simulink model "SMC_POS_SMC_Att"  (R2024b)
settings: Solver=FixedStepDiscrete  StartTime=0.0  StopTime=45  FixedStep=1/250  RelTol=1e-3
values from neighbouring files (symbols this model uses):
  a1 = 3.5524    [Parameter_SMC.m]
  a2 = 10.000    (= 10)    [Parameter_SMC.m]
  a3 = 8.1910    (= 8.191)    [Parameter_SMC.m]
  a4 = 2.7640    (= 2.764)    [Parameter_SMC.m]
  b3 = 0.6373    [Parameter_SMC.m]
  b4 = 0.0223    [Parameter_SMC.m]
  b_1x = 0.7426    [Parameter_SMC.m]
  b_1y = 0.5930    (= 0.593)    [Parameter_SMC.m]
  b_2x = 1.4305    [Parameter_SMC.m]
  b_2y = 1.0895    [Parameter_SMC.m]
  c_x = 0.2871    [Parameter_SMC.m]
  c_y = 0.3867    [Parameter_SMC.m]
  epsilon_1_a = 0.5    [Parameter_SMC.m]
  epsilon_1_b = 0.5    [Parameter_SMC.m]
  epsilon_2 = 0.5    [Parameter_SMC.m]
  epsilon_2_b = 0.5    [Parameter_SMC.m]
  g = 9.81    [Parameter_SMC.m]
  Jx = 0.005    [Parameter_SMC.m]
  Jy = 0.005    [Parameter_SMC.m]
  Jz = 0.009    [Parameter_SMC.m]
  K1 = 0.01    [Parameter_SMC.m]
  k1 = 0.001    [Parameter_SMC.m]
  K2 = 0    [Parameter_SMC.m]
  k2 = a1    (= 3.5524)    [Parameter_SMC.m]
  k3 = 0.1    [Parameter_SMC.m]
  k4 = 0.5000    (= 0.5)    [Parameter_SMC.m]
  k5 = 0.0388    [Parameter_SMC.m]
  k6 = Jx * a3 / (l * sqrt(8) * Tmax)    [Parameter_SMC.m]
  k7 = 0.3147    [Parameter_SMC.m]
  k8 = a4 * Jz / (4 * Qmax)    (= 0.12438)    [Parameter_SMC.m]
  k_ob = 1    [Parameter_SMC.m]
  l = 0.33/2    (= 0.165)    [Parameter_SMC.m]
  m = 0.8    [Parameter_SMC.m]
  PWM_max = 2000    [Parameter_SMC.m]
  PWM_min = 1000    [Parameter_SMC.m]
  Qmax = 0.05    [Parameter_SMC.m]
  Tmax = 4    [Parameter_SMC.m]
undefined symbols (not defined in the file or in its folder): d_1_x, DiscIntNeverNeededParam, k_1_a, k_1_b, k_2_a, k_2_b, K_4, Q_max, T_max
libraries: simulink x13, slpidlib x3
(part 1 of 2)
settings Model: Creator=user  LastModifiedBy=user

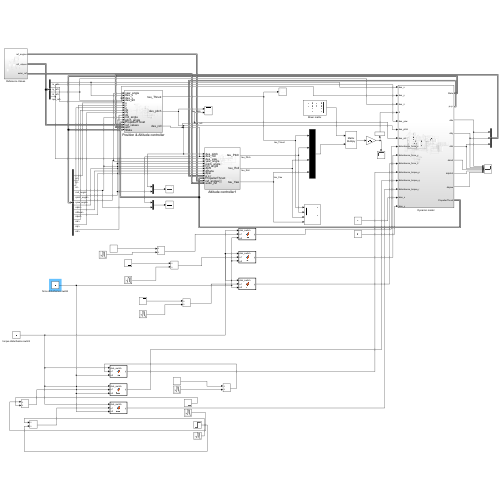
[thumbnail: Simulink's stored preview of the top-level diagram]
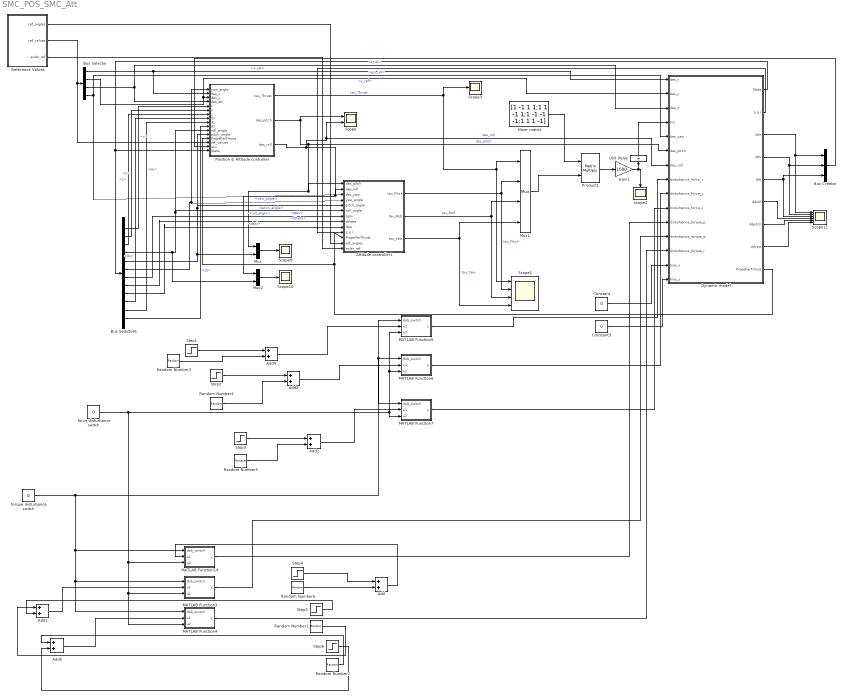
== system SMC_POS_SMC_Att ==
  Add{,1..5} (6 alike) : Sum
  Attitude controller1 : Subsystem
  Bus Creator : BusCreator  Inputs=3
  Bus Selector : BusSelector  OutputSignals=x_ref,y_ref,z_ref,psi_ref
  Bus Selector6 : BusSelector  OutputSignals=x,y,z,roll_angle,pitch_angle,yaw_angle,dphi,dtheta,dpsi,dx,dy,dz
  Constant : Constant  Value=0  SampleTime=-1
  Constant3 : Constant  Value=0  SampleTime=-1
  "Dynamic model " : Subsystem
  Gain1 : Gain  Gain=1000  OutDataTypeStr=double
  MATLAB Function14 : MATLAB Function  TreatAsAtomicUnit=on
  MATLAB Function3 : MATLAB Function  TreatAsAtomicUnit=on
  MATLAB Function4 : MATLAB Function  TreatAsAtomicUnit=on
  MATLAB Function5 : MATLAB Function  TreatAsAtomicUnit=on
  MATLAB Function6 : MATLAB Function  TreatAsAtomicUnit=on
  MATLAB Function7 : MATLAB Function  TreatAsAtomicUnit=on
  Mixer matrix : Constant  Value=[1 -1 1 1;1 1 -1 1;1 -1 -1 -1;1 1 1 -1]  OutDataTypeStr=Inherit: Inherit via back propagation
  Mux : Mux  Inputs=2
  Mux1 : Mux
  Mux2 : Mux  Inputs=2
  Position & Altitude controller : Subsystem
  Product1 : Product  Multiplication=Matrix(*)  RndMeth=Zero
  Random Number{1..6} (6 alike) : RandomNumber  Variance=0.1
  Reference Values : Subsystem
  Scope : Scope  NumInputPorts=2
  Scope1 : Scope  NumInputPorts=4
  Scope{2..3,9..10} (4 alike) : Scope
  Scope11 : Scope  NumInputPorts=6
  Step1 : Step  Time=0  After=15
  Step2 : Step  Time=0  After=-15
  Step3 : Step  Time=0  After=2
  Step4 : Step  Time=0
  Step5 : Step  Time=0  After=-0.5
  Step6 : Step  Time=0  After=5
  Unit Delay : UnitDelay  SampleTime=-1  HasFrameUpgradeWarning=on
  force disturbance switch : Constant  Value=0  SampleTime=-1
  torque disturbance switch : Constant  Value=0  SampleTime=-1
  wires:
  "Dynamic model "/5(ddz) -> Bus Creator/3, Scope11/3
  Constant3/1 -> "Dynamic model "/15(bias_y)
  Bus Selector6/12 -> Position & Altitude controller/10(dz)  "<dz>"
  "Dynamic model "/8(ddyaw) -> Scope11/6
  Product1/1 -> Gain1/1
  Mux/1 -> Scope9/1
  Mixer matrix/1 -> Product1/1
  Position & Altitude controller/2(des_pitch) -> Scope/1, Mux/1, Attitude controller1/1(des_pitch), "Dynamic model "/6(des_pitch)  "des_pitch"
  "Dynamic model "/2(p q r) -> Attitude controller1/10(p q r)
  "Dynamic model "/1(State) -> Bus Selector6/1, Position & Altitude controller/16(State)
  Bus Selector6/11 -> Position & Altitude controller/9(dy)  "<dy>"
  Attitude controller1/3(tau_Yaw) -> Mux1/4, Scope1/4  "tau_Yaw"
  Bus Selector6/2 -> Position & Altitude controller/6(y)  "<y>"
  "Dynamic model "/9(PropellerThrust) -> Position & Altitude controller/13(PropellerThrust), Attitude controller1/11(PropellerThrust)
  Attitude controller1/1(tau_Pitch) -> Mux1/2, Scope1/2  "tau_Pitch"
  Constant/1 -> "Dynamic model "/14(bias_x)
  "Dynamic model "/4(ddy) -> Bus Creator/2, Scope11/2
  Bus Selector6/1 -> Position & Altitude controller/5(x)  "<x>"
  Mux2/1 -> Scope10/1
  Bus Selector6/9 -> Attitude controller1/9(dpsi)  "<dpsi>"
  Bus Selector6/5 -> Position & Altitude controller/12(pitch_angle), Attitude controller1/5(pitch_angle), Mux/2  "<pitch_angle>"
  Gain1/1 -> Scope2/1, Unit Delay/1
  Bus Selector6/10 -> Position & Altitude controller/8(dx)  "<dx>"
  Bus Selector6/6 -> Position & Altitude controller/1(yaw_angle), Attitude controller1/4(yaw_angle)  "<yaw_angle>"
  Position & Altitude controller/1(tau_Thrust) -> Scope3/1, Mux1/1, Scope1/1  "tau_Thrust"
  Bus Selector6/4 -> Mux2/2, Position & Altitude controller/11(roll_angle), Attitude controller1/6(roll_angle)  "<roll_angle>"
  "Dynamic model "/6(ddroll) -> Scope11/4
  "Dynamic model "/7(ddpitch) -> Scope11/5
  Bus Selector6/8 -> Attitude controller1/8(dtheta)  "<dtheta>"
  Bus Selector6/7 -> Attitude controller1/7(dphi)  "<dphi>"
  Attitude controller1/2(tau_Roll) -> Mux1/3, Scope1/3  "tau_Roll"
  Position & Altitude controller/3(des_roll) -> Mux2/1, Attitude controller1/2(des_roll), "Dynamic model "/7(des_roll), Scope/2  "des_roll"
  "Dynamic model "/3(ddx) -> Bus Creator/1, Scope11/1
  Bus Selector6/3 -> Position & Altitude controller/7(z)  "<z>"
  Mux1/1 -> Product1/2
  Reference Values/2(ref_values) -> Position & Altitude controller/14(ref_values), Bus Selector/1
  Bus Selector/1 -> "Dynamic model "/1(des_x), Position & Altitude controller/2(des_x)  "<x_ref>"
  Bus Selector/2 -> "Dynamic model "/2(des_y), Position & Altitude controller/3(des_y)  "<y_ref>"
  Bus Selector/3 -> Position & Altitude controller/4(des_alt), "Dynamic model "/3(des_z)  "<z_ref>"
  Bus Selector/4 -> Attitude controller1/3(des_yaw), "Dynamic model "/5(des_yaw)  "<psi_ref>"
  Reference Values/1(ref_angles) -> Attitude controller1/12(ref_angles)
  Reference Values/3(euler_ref) -> Attitude controller1/13(euler_ref)
  Bus Creator/1 -> Position & Altitude controller/15(acc)
  Unit Delay/1 -> "Dynamic model "/4(In1)
  Random Number1/1 -> Add1/1
  Add4/1 -> MATLAB Function5/2(u1)
  torque disturbance switch/1 -> MATLAB Function5/1(dob_switch), MATLAB Function7/1(dob_switch), MATLAB Function6/1(dob_switch), MATLAB Function14/1(dob_switch), MATLAB Function4/1(dob_switch), MATLAB Function3/1(dob_switch)
  Step3/1 -> Add2/1
  Step6/1 -> Add5/2
  Step2/1 -> Add3/1
  Add2/1 -> MATLAB Function7/2(u1)
  Random Number2/1 -> Add5/1
  Step4/1 -> Add/1
  Random Number6/1 -> Add/2
  Add5/1 -> MATLAB Function4/2(u1)
  Random Number3/1 -> Add4/2
  Random Number4/1 -> Add3/2
  Add1/1 -> MATLAB Function3/2(u1)
  Random Number5/1 -> Add2/2
  force disturbance switch/1 -> MATLAB Function5/3(u2), MATLAB Function6/3(u2), MATLAB Function7/3(u2), MATLAB Function4/3(u2), MATLAB Function3/3(u2), MATLAB Function14/3(u2)
  Step5/1 -> Add1/2
  Add3/1 -> MATLAB Function6/2(u1)
  Step1/1 -> Add4/1
  Add/1 -> MATLAB Function14/2(u1)
  MATLAB Function5/1(y) -> "Dynamic model "/8(disturbance_force_x)
  MATLAB Function6/1(y) -> "Dynamic model "/9(disturbance_force_y)
  MATLAB Function7/1(y) -> "Dynamic model "/10(disturbance_force_z)
  MATLAB Function14/1(y) -> "Dynamic model "/11(disturbance_torque_p)
  MATLAB Function3/1(y) -> "Dynamic model "/12(disturbance_torque_q)
  MATLAB Function4/1(y) -> "Dynamic model "/13(disturbance_torque_r)

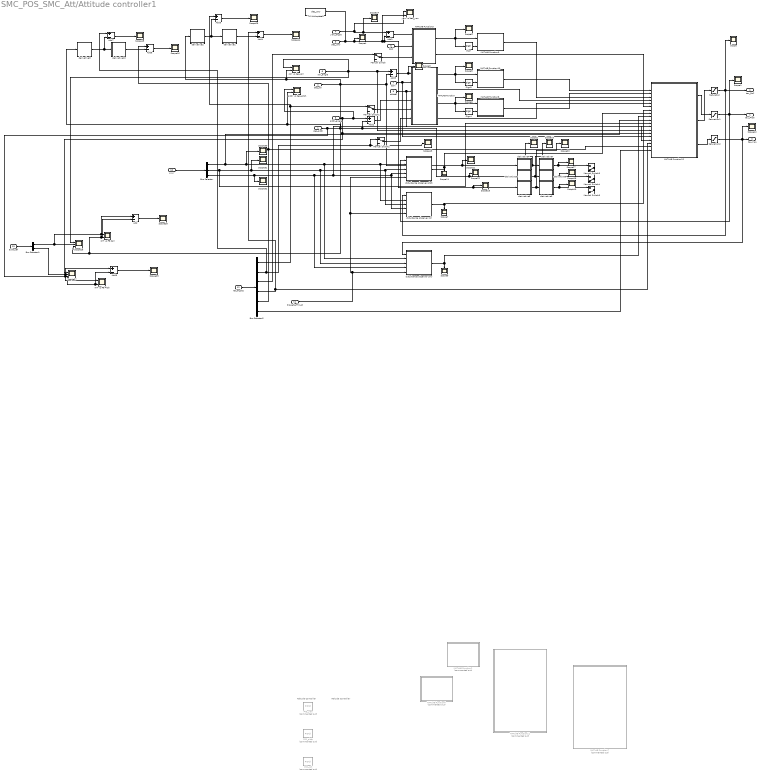
== system SMC_POS_SMC_Att/Attitude controller1 ==
  note: Attitude Controller
  note: Attitude Controller
  des_pitch : Inport
  des_roll : Inport  Port=2
  des_yaw : Inport  Port=3
  yaw_angle : Inport  Port=4
  pitch_angle : Inport  Port=5
  roll_angle : Inport  Port=6
  dphi : Inport  Port=7
  dtheta : Inport  Port=8
  dpsi : Inport  Port=9
  p q r : Inport  Port=10
  PropellerThrust : Inport  Port=11
  ref_angles : Inport  Port=12
  euler_ref : Inport  Port=13
  Add{,1..8} (9 alike) : Sum  Inputs=+-
  Bus Selector : BusSelector  OutputSignals=p,q,r
  Bus Selector1 : BusSelector  OutputSignals=phi_ref,theta_ref
  Bus Selector2 : BusSelector  OutputSignals=dphi_ref,dtheta_ref,dpsi_ref,ddphi_ref,ddtheta_ref,ddpsi_ref
  MATLAB Function : MATLAB Function  TreatAsAtomicUnit=on
  MATLAB Function10 : MATLAB Function  TreatAsAtomicUnit=on
  MATLAB Function11 : MATLAB Function  Commented=on  TreatAsAtomicUnit=on
  MATLAB Function12 : MATLAB Function  TreatAsAtomicUnit=on
  MATLAB Function3 : MATLAB Function  TreatAsAtomicUnit=on
  MATLAB Function5 : MATLAB Function  Commented=on  TreatAsAtomicUnit=on
  MATLAB Function6 : MATLAB Function  Commented=on  TreatAsAtomicUnit=on
  MATLAB Function7 : MATLAB Function  Commented=on  TreatAsAtomicUnit=on
  MATLAB Function8 : MATLAB Function  TreatAsAtomicUnit=on
  MATLAB Function9 : MATLAB Function  TreatAsAtomicUnit=on
  Manual Switch : ManualSwitch
  Manual Switch1 : ManualSwitch
  Manual Switch2 : ManualSwitch
  Manual Switch3 : ManualSwitch  CurrentSetting=0
  Manual Switch4 : ManualSwitch  CurrentSetting=0
  Manual Switch5 : ManualSwitch  CurrentSetting=0
  NIT vs FB Pitch : Scope  NumInputPorts=2
  NIT vs FB Roll : Scope  NumInputPorts=2
  PID_pitch : slpidlib/PID Controller  Commented=on  Controller=PID  Form=Parallel  TimeDomain=Continuous-time  UseExternalTs=off  SampleTime=-1  IntegratorMethod=Backward Euler  FilterMethod=Forward Euler  ControllerParametersSource=internal  P=0.027  I=0.005  UseKiTs=off  D=0.0145948093220339  UseExternalDerivativeSource=off  N=50  UseFilter=on  TunerSelectOption=Transfer Function Based (PID Tuner App)  InitialConditionSource=internal  InitialConditionForIntegrator=0  InitialConditionForFilter=0  DifferentiatorICPrevScaledInput=0  ExternalReset=level  TrackingMode=off  Kt=1  LimitOutput=on  SatLimitsSource=internal  UpperSaturationLimit=0.05  LowerSaturationLimit=-0.05  LinearizeAsGain=off  AntiWindupMode=none  Kb=1  LimitIntegrator=off  UpperIntegratorSaturationLimit=inf  LowerIntegratorSaturationLimit=-inf  POutMin=[]  POutMax=[]  IOutMin=[]  IOutMax=[]  DOutMin=[]  DOutMax=[]  NOutMin=[]  NOutMax=[]  SumOutMin=[]  SumOutMax=[]  SaturationOutMin=[]  SaturationOutMax=[]  PParamMin=[]  PParamMax=[]  IParamMin=[]  IParamMax=[]  DParamMin=[]  DParamMax=[]  NParamMin=[]  NParamMax=[]  KbParamMin=[]  KbParamMax=[]  KtParamMin=[]  KtParamMax=[]  KbOutMin=[]  KbOutMax=[]  KtOutMin=[]  KtOutMax=[]  IntegratorOutMin=[]  IntegratorOutMax=[]  FilterOutMin=[]  FilterOutMax=[]  SumI1OutMin=[]  SumI1OutMax=[]  SumI2OutMin=[]  SumI2OutMax=[]  SumI3OutMin=[]  SumI3OutMax=[]  SumI4OutMin=[]  SumI4OutMax=[]  SumDOutMin=[]  SumDOutMax=[]  DifferentiatorOutMin=[]  DifferentiatorOutMax=[]  FilterDiffOutCoefMin=[]  FilterDiffOutCoefMax=[]  ReciprocalOutMin=[]  ReciprocalOutMax=[]  SumDenOutMin=[]  SumDenOutMax=[]  SumNumOutMin=[]  SumNumOutMax=[]  DivideOutMin=[]  DivideOutMax=[]  UdiffTsProdOutMin=[]  UdiffTsProdOutMax=[]  NTsProdOutMin=[]  NTsProdOutMax=[]  UintegralTsProdOutMin=[]  UintegralTsProdOutMax=[]  UngainTsProdOutMin=[]  UngainTsProdOutMax=[]  ClampingZeroOutDataTypeStr=Inherit: Inherit via back propagation  ClampingZeroOutMin=[]  ClampingZeroOutMax=[]  FilterDenConstantOutDataTypeStr=Inherit: Inherit via back propagation  FilterDenConstantOutMin=[]  FilterDenConstantOutMax=[]  PCopyOutDataTypeStr=Inherit: Inherit via back propagation  PCopyOutMin=[]  PCopyOutMax=[]  NCopyOutDataTypeStr=Inherit: Inherit via back propagation  NCopyOutMin=[]  NCopyOutMax=[]  IntegratorContinuousStateAttributes=''  IntegratorStateMustResolveToSignalObject=off  IntegratorRTWStateStorageClass=Auto  FilterContinuousStateAttributes=''  FilterStateMustResolveToSignalObject=off  FilterRTWStateStorageClass=Auto  ParallelPVariant=InternalParameters  IdealPVariant=Disabled  IVariant=InternalParameters  DVariant=InternalParameters  IntegratorVariant=Continuous  SatVariant=Enabled  AWVariant=Passthrough  PCopyVariant=Disabled  TRVariant=Disabled  FdbkBlocksVariant=Forward  IdealPFdbkVariant=Disabled  SatFdbkVariant=Disabled  DerivativeFilterVariant=ContFilter  NVariant=InternalParameters  NCopyVariant=Disabled  FilterICVariant=InternalICsFilter  IntegratorICVariant=InternalICs  ExternalResetVariant=ExternalReset  TRSumVariant=Passthrough  SumFdbkVariant=Disabled  SumVariant=Sum_PID  TsampFilterVariant=InternalTs  TsampNgainVariant=Passthrough  TsampIntegralVariant=Disabled_SignalSpec  ExternalSaturationOutDataTypeStr=Inherit: Same as second input  DerivativeSourceVariant=ErrorSignal  PreIntVariant=InternalPreInt
  PID_roll : slpidlib/PID Controller  Commented=on  Controller=PID  Form=Parallel  TimeDomain=Continuous-time  UseExternalTs=off  SampleTime=-1  IntegratorMethod=Backward Euler  FilterMethod=Forward Euler  ControllerParametersSource=internal  P=0.03  I=0.005  UseKiTs=off  D=0.015  UseExternalDerivativeSource=off  N=100  UseFilter=on  TunerSelectOption=Transfer Function Based (PID Tuner App)  InitialConditionSource=internal  InitialConditionForIntegrator=0  InitialConditionForFilter=0  DifferentiatorICPrevScaledInput=0  ExternalReset=level  TrackingMode=off  Kt=1  LimitOutput=on  SatLimitsSource=internal  UpperSaturationLimit=0.05  LowerSaturationLimit=-0.05  LinearizeAsGain=off  AntiWindupMode=none  Kb=1  LimitIntegrator=off  UpperIntegratorSaturationLimit=inf  LowerIntegratorSaturationLimit=-inf  POutMin=[]  POutMax=[]  IOutMin=[]  IOutMax=[]  DOutMin=[]  DOutMax=[]  NOutMin=[]  NOutMax=[]  SumOutMin=[]  SumOutMax=[]  SaturationOutMin=[]  SaturationOutMax=[]  PParamMin=[]  PParamMax=[]  IParamMin=[]  IParamMax=[]  DParamMin=[]  DParamMax=[]  NParamMin=[]  NParamMax=[]  KbParamMin=[]  KbParamMax=[]  KtParamMin=[]  KtParamMax=[]  KbOutMin=[]  KbOutMax=[]  KtOutMin=[]  KtOutMax=[]  IntegratorOutMin=[]  IntegratorOutMax=[]  FilterOutMin=[]  FilterOutMax=[]  SumI1OutMin=[]  SumI1OutMax=[]  SumI2OutMin=[]  SumI2OutMax=[]  SumI3OutMin=[]  SumI3OutMax=[]  SumI4OutMin=[]  SumI4OutMax=[]  SumDOutMin=[]  SumDOutMax=[]  DifferentiatorOutMin=[]  DifferentiatorOutMax=[]  FilterDiffOutCoefMin=[]  FilterDiffOutCoefMax=[]  ReciprocalOutMin=[]  ReciprocalOutMax=[]  SumDenOutMin=[]  SumDenOutMax=[]  SumNumOutMin=[]  SumNumOutMax=[]  DivideOutMin=[]  DivideOutMax=[]  UdiffTsProdOutMin=[]  UdiffTsProdOutMax=[]  NTsProdOutMin=[]  NTsProdOutMax=[]  UintegralTsProdOutMin=[]  UintegralTsProdOutMax=[]  UngainTsProdOutMin=[]  UngainTsProdOutMax=[]  ClampingZeroOutDataTypeStr=Inherit: Inherit via back propagation  ClampingZeroOutMin=[]  ClampingZeroOutMax=[]  FilterDenConstantOutDataTypeStr=Inherit: Inherit via back propagation  FilterDenConstantOutMin=[]  FilterDenConstantOutMax=[]  PCopyOutDataTypeStr=Inherit: Inherit via back propagation  PCopyOutMin=[]  PCopyOutMax=[]  NCopyOutDataTypeStr=Inherit: Inherit via back propagation  NCopyOutMin=[]  NCopyOutMax=[]  IntegratorContinuousStateAttributes=''  IntegratorStateMustResolveToSignalObject=off  IntegratorRTWStateStorageClass=Auto  FilterContinuousStateAttributes=''  FilterStateMustResolveToSignalObject=off  FilterRTWStateStorageClass=Auto  ParallelPVariant=InternalParameters  IdealPVariant=Disabled  IVariant=InternalParameters  DVariant=InternalParameters  IntegratorVariant=Continuous  SatVariant=Enabled  AWVariant=Passthrough  PCopyVariant=Disabled  TRVariant=Disabled  FdbkBlocksVariant=Forward  IdealPFdbkVariant=Disabled  SatFdbkVariant=Disabled  DerivativeFilterVariant=ContFilter  NVariant=InternalParameters  NCopyVariant=Disabled  FilterICVariant=InternalICsFilter  IntegratorICVariant=InternalICs  ExternalResetVariant=ExternalReset  TRSumVariant=Passthrough  SumFdbkVariant=Disabled  SumVariant=Sum_PID  TsampFilterVariant=InternalTs  TsampNgainVariant=Passthrough  TsampIntegralVariant=Disabled_SignalSpec  ExternalSaturationOutDataTypeStr=Inherit: Same as second input  DerivativeSourceVariant=ErrorSignal  PreIntVariant=InternalPreInt
  PID_yaw : slpidlib/PID Controller  Commented=on  Controller=PID  Form=Parallel  TimeDomain=Continuous-time  UseExternalTs=off  SampleTime=-1  IntegratorMethod=Backward Euler  FilterMethod=Forward Euler  ControllerParametersSource=internal  P=0.08024000000000001  I=0.005  UseKiTs=off  D=0.075  UseExternalDerivativeSource=off  N=100  UseFilter=on  TunerSelectOption=Transfer Function Based (PID Tuner App)  InitialConditionSource=internal  InitialConditionForIntegrator=0  InitialConditionForFilter=0  DifferentiatorICPrevScaledInput=0  ExternalReset=level  TrackingMode=off  Kt=1  LimitOutput=on  SatLimitsSource=internal  UpperSaturationLimit=0.1  LowerSaturationLimit=-0.1  LinearizeAsGain=off  AntiWindupMode=none  Kb=1  LimitIntegrator=off  UpperIntegratorSaturationLimit=inf  LowerIntegratorSaturationLimit=-inf  POutMin=[]  POutMax=[]  IOutMin=[]  IOutMax=[]  DOutMin=[]  DOutMax=[]  NOutMin=[]  NOutMax=[]  SumOutMin=[]  SumOutMax=[]  SaturationOutMin=[]  SaturationOutMax=[]  PParamMin=[]  PParamMax=[]  IParamMin=[]  IParamMax=[]  DParamMin=[]  DParamMax=[]  NParamMin=[]  NParamMax=[]  KbParamMin=[]  KbParamMax=[]  KtParamMin=[]  KtParamMax=[]  KbOutMin=[]  KbOutMax=[]  KtOutMin=[]  KtOutMax=[]  IntegratorOutMin=[]  IntegratorOutMax=[]  FilterOutMin=[]  FilterOutMax=[]  SumI1OutMin=[]  SumI1OutMax=[]  SumI2OutMin=[]  SumI2OutMax=[]  SumI3OutMin=[]  SumI3OutMax=[]  SumI4OutMin=[]  SumI4OutMax=[]  SumDOutMin=[]  SumDOutMax=[]  DifferentiatorOutMin=[]  DifferentiatorOutMax=[]  FilterDiffOutCoefMin=[]  FilterDiffOutCoefMax=[]  ReciprocalOutMin=[]  ReciprocalOutMax=[]  SumDenOutMin=[]  SumDenOutMax=[]  SumNumOutMin=[]  SumNumOutMax=[]  DivideOutMin=[]  DivideOutMax=[]  UdiffTsProdOutMin=[]  UdiffTsProdOutMax=[]  NTsProdOutMin=[]  NTsProdOutMax=[]  UintegralTsProdOutMin=[]  UintegralTsProdOutMax=[]  UngainTsProdOutMin=[]  UngainTsProdOutMax=[]  ClampingZeroOutDataTypeStr=Inherit: Inherit via back propagation  ClampingZeroOutMin=[]  ClampingZeroOutMax=[]  FilterDenConstantOutDataTypeStr=Inherit: Inherit via back propagation  FilterDenConstantOutMin=[]  FilterDenConstantOutMax=[]  PCopyOutDataTypeStr=Inherit: Inherit via back propagation  PCopyOutMin=[]  PCopyOutMax=[]  NCopyOutDataTypeStr=Inherit: Inherit via back propagation  NCopyOutMin=[]  NCopyOutMax=[]  IntegratorContinuousStateAttributes=''  IntegratorStateMustResolveToSignalObject=off  IntegratorRTWStateStorageClass=Auto  FilterContinuousStateAttributes=''  FilterStateMustResolveToSignalObject=off  FilterRTWStateStorageClass=Auto  ParallelPVariant=InternalParameters  IdealPVariant=Disabled  IVariant=InternalParameters  DVariant=InternalParameters  IntegratorVariant=Continuous  SatVariant=Enabled  AWVariant=Passthrough  PCopyVariant=Disabled  TRVariant=Disabled  FdbkBlocksVariant=Forward  IdealPFdbkVariant=Disabled  SatFdbkVariant=Disabled  DerivativeFilterVariant=ContFilter  NVariant=InternalParameters  NCopyVariant=Disabled  FilterICVariant=InternalICsFilter  IntegratorICVariant=InternalICs  ExternalResetVariant=ExternalReset  TRSumVariant=Passthrough  SumFdbkVariant=Disabled  SumVariant=Sum_PID  TsampFilterVariant=InternalTs  TsampNgainVariant=Passthrough  TsampIntegralVariant=Disabled_SignalSpec  ExternalSaturationOutDataTypeStr=Inherit: Same as second input  DerivativeSourceVariant=ErrorSignal  PreIntVariant=InternalPreInt
  Saturation : Saturate  UpperLimit=0.05  LowerLimit=-0.05
  Saturation1 : Saturate  UpperLimit=0.05  LowerLimit=-0.05
  Saturation2 : Saturate  UpperLimit=0.1  LowerLimit=-0.1
  Scope{,1..25,28..32} (31 alike) : Scope
  Scope26 : Scope  NumInputPorts=3
  Scope27 : Scope  NumInputPorts=3
  Sign : Signum
  Sign4 : Signum
  Sign5 : Signum
  To Workspace3 : ToWorkspace  VariableName=des_yaw  SampleTime=-1
      settings: Save2DSignal=2-D array (concatenate along first dimension)
  derivative1 : Subsystem
  derivative10 : Subsystem
  derivative2 : Subsystem
  derivative3 : Subsystem
  derivative4 : Subsystem
  derivative5 : Subsystem
  derivative6 : Subsystem
  derivative7 : Subsystem
  derivative8 : Subsystem
  derivative9 : Subsystem
  disturbance observer pitch : Subsystem
  disturbance observer roll : Subsystem
  disturbance observer yaw : Subsystem
  pitch vs des_pitch : Scope  NumInputPorts=2
  roll vs des_roll : Scope  NumInputPorts=2
  yaw vs des_yaw : Scope  NumInputPorts=2
  tau_Pitch : Outport
  tau_Roll : Outport  Port=2
  tau_Yaw : Outport  Port=3
  wires:
  yaw_angle/1 -> Scope24/1, Add1/1, yaw vs des_yaw/1  "yaw_angle"
  des_yaw/1 -> To Workspace3/1, Scope4/1, yaw vs des_yaw/2, Scope23/1, derivative6/1(In1), Add1/2  "des_yaw"
  Saturation/1 -> Scope/1, tau_Roll/1, disturbance observer roll/1(tau_Roll)
  Saturation2/1 -> Scope12/1, disturbance observer yaw/1(tau_Yaw), tau_Yaw/1
  Add1/1 -> MATLAB Function3/1(error)  "yaw_error"
  MATLAB Function/2(error_dphi) -> MATLAB Function12/4(error_dphi)
  MATLAB Function/1(s_phi) -> Scope5/1, Sign5/1, MATLAB Function10/1(s)
  MATLAB Function/4(error_dtheta) -> MATLAB Function12/5(error_dtheta)
  MATLAB Function/3(s_theta) -> Scope6/1, Sign4/1, MATLAB Function8/1(s)
  dtheta/1 -> MATLAB Function12/16(dtheta), MATLAB Function/3(dtheta)
  dphi/1 -> MATLAB Function12/15(dphi), MATLAB Function/2(dphi)
  Add3/1 -> Scope8/1, MATLAB Function/1(error_phi)  "roll_error"
  Add2/1 -> MATLAB Function/4(error_theta)  "pitch_error"
  MATLAB Function3/2(error_dpsi) -> MATLAB Function12/6(error_dpsi)
  MATLAB Function3/1(s_psi) -> Scope3/1, Sign/1, MATLAB Function9/1(s)
  dpsi/1 -> MATLAB Function3/2(dpsi)
  p q r/1 -> Bus Selector/1
  Bus Selector/1 -> MATLAB Function12/10(p), Scope30/1, disturbance observer roll/2("p "), disturbance observer pitch/2("p "), disturbance observer yaw/2("p ")  "<p>"
  Bus Selector/2 -> disturbance observer pitch/3(q), disturbance observer roll/3(q), disturbance observer yaw/3(q), Scope31/1, MATLAB Function12/11(q)  "<q>"
  Bus Selector/3 -> MATLAB Function12/12(r), disturbance observer pitch/4(r), disturbance observer roll/4(r), disturbance observer yaw/4(r), Scope32/1  "<r>"
  disturbance observer pitch/1(d_ob) -> MATLAB Function12/8(d_ob_theta), Scope11/1
  disturbance observer roll/1(d_ob) -> MATLAB Function12/7(d_ob_phi), Scope7/1
  disturbance observer yaw/1(d_ob) -> Scope9/1, MATLAB Function12/9(d_ob_psi)
  Manual Switch/1 -> MATLAB Function3/3(des_dpsi)
  Manual Switch1/1 -> MATLAB Function/5(des_dphi)
  Manual Switch2/1 -> MATLAB Function/6(des_dtheta)
  Saturation1/1 -> disturbance observer pitch/1(tau_Pitch), tau_Pitch/1, Scope1/1
  Sign/1 -> MATLAB Function9/2(sgn)
  Sign4/1 -> MATLAB Function8/2(sgn)
  Sign5/1 -> MATLAB Function10/2(sgn)
  MATLAB Function10/1(sat_phi) -> MATLAB Function12/1(sat_phi)
  MATLAB Function8/1(sat_theta) -> MATLAB Function12/2(sat_theta)
  MATLAB Function9/1(sat_psi) -> MATLAB Function12/3(sat_psi)
  derivative4/1(Out1) -> Scope2/1, derivative7/1(In1)
  derivative5/1(Out1) -> Scope10/1, derivative8/1(In1)
  derivative6/1(Out1) -> Scope20/1, derivative9/1(In1)
  derivative7/1(Out1) -> Scope17/1, Manual Switch3/1
  derivative8/1(Out1) -> Scope18/1, Manual Switch4/1
  derivative9/1(Out1) -> Scope19/1, Manual Switch5/1
  MATLAB Function12/3(tau_yaw) -> Saturation2/1
  MATLAB Function12/1(tau_pitch) -> Saturation1/1
  MATLAB Function12/2(tau_roll) -> Saturation/1
  PropellerThrust/1 -> disturbance observer yaw/5(PropellerThrust), disturbance observer pitch/5(PropellerThrust), disturbance observer roll/5(PropellerThrust)
  ref_angles/1 -> Bus Selector2/1
  Bus Selector2/1 -> Add5/1, Manual Switch1/1  "<dphi_ref>"
  Bus Selector2/3 -> Manual Switch/1  "<dpsi_ref>"
  Bus Selector2/6 -> MATLAB Function12/19(des_ddpsi)  "<ddpsi_ref>"
  derivative3/1(Out1) -> Add7/2, derivative10/1(des_roll)  "d_theta_des"
  Add4/1 -> Scope14/1  "dd_phi ref-des"
  Add7/1 -> Scope15/1  "d_theta ref-des"
  derivative2/1(Out1) -> Add5/2, derivative1/1(des_roll)  "d_phi_des"
  derivative1/1(Out1) -> Add4/2  "dd_phi_des"
  Bus Selector2/2 -> Add7/1, Manual Switch2/1, Scope13/1  "<dtheta_ref>"
  Add5/1 -> Scope25/1  "d_phi ref-des"
  Bus Selector2/4 -> Add4/1, MATLAB Function12/17(des_ddphi)  "<ddphi_ref>"
  derivative10/1(Out1) -> Add6/2  "dd_theta_des"
  Add6/1 -> Scope16/1  "dd_theta ref-des"
  Bus Selector2/5 -> Add6/1, MATLAB Function12/18(des_ddtheta)  "<ddtheta_ref>"
  euler_ref/1 -> Bus Selector1/1
  pitch_angle/1 -> pitch vs des_pitch/1, Add2/1, Scope27/1, MATLAB Function12/14(theta)  "pitch_angle"
  Bus Selector1/1 -> Scope26/2, Add/1, NIT vs FB Roll/1  "<phi_ref>"
  Bus Selector1/2 -> NIT vs FB Pitch/1, Scope27/2, Add8/1  "<theta_ref>"
  roll_angle/1 -> roll vs des_roll/1, Scope26/1, MATLAB Function12/13(phi), Add3/1  "roll _angle"
  des_pitch/1 -> Add8/2, NIT vs FB Pitch/2, Scope27/3, derivative3/1(des_roll), pitch vs des_pitch/2, Scope22/1, derivative5/1(In1), Add2/2  "des_pitch"
  des_roll/1 -> Add/2, NIT vs FB Roll/2, Scope26/3, derivative2/1(des_roll), roll vs des_roll/2, Scope21/1, derivative4/1(In1), Add3/2  "des_roll"
  Add/1 -> Scope28/1  "NIT - FB Roll"
  Add8/1 -> Scope29/1  "NIT - FB Pitch"

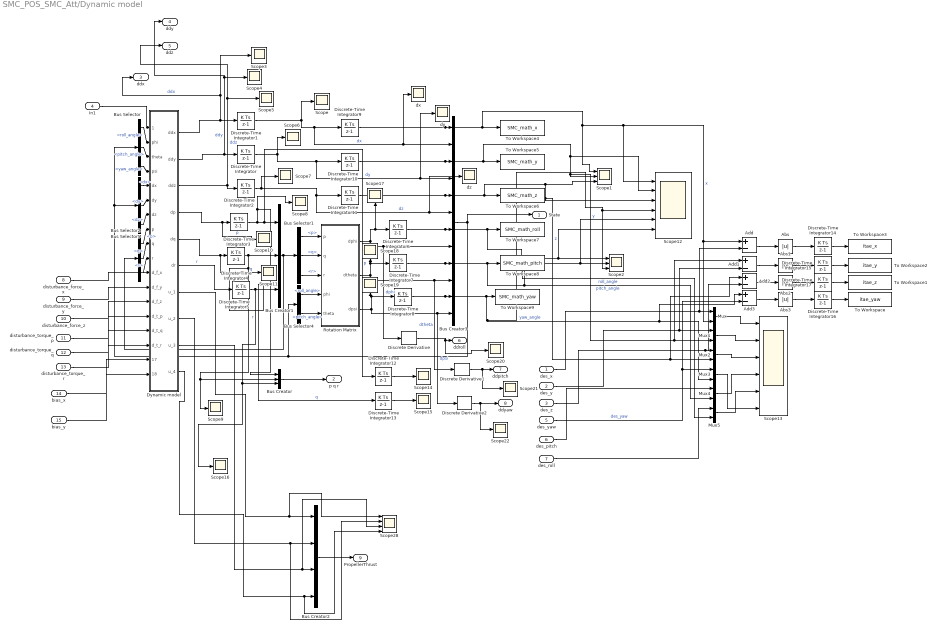
== system SMC_POS_SMC_Att/Dynamic model  ==
  des_x : Inport
  des_y : Inport  Port=2
  des_z : Inport  Port=3
  In1 : Inport  Port=4
  des_yaw : Inport  Port=5
  des_pitch : Inport  Port=6
  des_roll : Inport  Port=7
  disturbance_force_x : Inport  Port=8
  disturbance_force_y : Inport  Port=9
  disturbance_force_z : Inport  Port=10
  disturbance_torque_p : Inport  Port=11
  disturbance_torque_q : Inport  Port=12
  disturbance_torque_r : Inport  Port=13
  bias_x : Inport  Port=14
  bias_y : Inport  Port=15
  Abs{,1..3} (4 alike) : Abs  SaturateOnIntegerOverflow=off
  Add{,1..3} (4 alike) : Sum  Inputs=+-
  Bus Creator : BusCreator  Inputs=3
  Bus Creator1 : BusCreator  Inputs=3
  Bus Creator2 : BusCreator  Inputs=4
  Bus Creator3 : BusCreator  Inputs=12
  Bus Selector : BusSelector  OutputSignals=roll_angle,pitch_angle,yaw_angle
  Bus Selector1 : BusSelector  OutputSignals=p,q,r
  Bus Selector2 : BusSelector  OutputSignals=p,q,r
  Bus Selector4 : BusSelector  OutputSignals=roll_angle,pitch_angle
  Bus Selector5 : BusSelector  OutputSignals=dx,dy,dz
  Discrete Derivative : simulink/Discrete/Discrete Derivative  gainval=1.0  ICPrevScaledInput=0.0  OutMin=[]  OutMax=[]  OutDataType=fixdt(1, 16)  OutScaling=2^-10  DoSatur=off
  Discrete Derivative1 : simulink/Discrete/Discrete Derivative  gainval=1.0  ICPrevScaledInput=0.0  OutMin=[]  OutMax=[]  OutDataType=fixdt(1, 16)  OutScaling=2^-10  DoSatur=off
  Discrete Derivative2 : simulink/Discrete/Discrete Derivative  gainval=1.0  ICPrevScaledInput=0.0  OutMin=[]  OutMax=[]  OutDataType=fixdt(1, 16)  OutScaling=2^-10  DoSatur=off
  Discrete-Time Integrator{,1..17} (18 alike) : DiscreteIntegrator  SampleTime=-1  ICPrevOutput=DiscIntNeverNeededParam  ICPrevScaledInput=DiscIntNeverNeededParam
  Dynamic model : MATLAB Function  TreatAsAtomicUnit=on
  Mux{,1..5} (6 alike) : Mux  Inputs=2
  Rotation Matrix : MATLAB Function  TreatAsAtomicUnit=on
  Scope{,3..11,14..22} (19 alike) : Scope
  Scope1 : Scope  NumInputPorts=3
  Scope12 : Scope  NumInputPorts=6
  Scope13 : Scope  NumInputPorts=6
  Scope2 : Scope  NumInputPorts=3
  Scope28 : Scope  NumInputPorts=4
  To Workspace : ToWorkspace  VariableName=itae_yaw  SampleTime=-1
      settings: Save2DSignal=2-D array (concatenate along first dimension)
  To Workspace1 : ToWorkspace  VariableName=itae_z  SampleTime=-1
      settings: Save2DSignal=2-D array (concatenate along first dimension)
  To Workspace2 : ToWorkspace  VariableName=itae_y  SampleTime=-1
      settings: Save2DSignal=2-D array (concatenate along first dimension)
  To Workspace3 : ToWorkspace  VariableName=itae_x  SampleTime=-1
      settings: Save2DSignal=2-D array (concatenate along first dimension)
  To Workspace4 : ToWorkspace  VariableName=SMC_math_x  SampleTime=-1
      settings: Save2DSignal=2-D array (concatenate along first dimension)
  To Workspace5 : ToWorkspace  VariableName=SMC_math_y  SampleTime=-1
      settings: Save2DSignal=2-D array (concatenate along first dimension)
  To Workspace6 : ToWorkspace  VariableName=SMC_math_z  SampleTime=-1
      settings: Save2DSignal=2-D array (concatenate along first dimension)
  To Workspace7 : ToWorkspace  VariableName=SMC_math_roll  SampleTime=-1
      settings: Save2DSignal=2-D array (concatenate along first dimension)
  To Workspace8 : ToWorkspace  VariableName=SMC_math_pitch  SampleTime=-1
      settings: Save2DSignal=2-D array (concatenate along first dimension)
  To Workspace9 : ToWorkspace  VariableName=SMC_math_yaw  SampleTime=-1
      settings: Save2DSignal=2-D array (concatenate along first dimension)
  dx : Scope
  dy : Scope
  dz : Scope
  State : Outport
  p q r : Outport  Port=2
  ddx : Outport  Port=3
  ddy : Outport  Port=4
  ddz : Outport  Port=5
  ddroll : Outport  Port=6
  ddpitch : Outport  Port=7
  ddyaw : Outport  Port=8
  PropellerThrust : Outport  Port=9
  wires:
  Discrete-Time Integrator2/1 -> Scope7/1, Discrete-Time Integrator11/1, dz/1, Bus Creator3/6  "dz"
  Bus Selector4/1 -> Rotation Matrix/4(phi)  "<roll_angle>"
  Bus Selector5/1 -> Dynamic model/5(dx)  "<dx>"
  Dynamic model/3(ddz) -> Discrete-Time Integrator2/1, Scope5/1, ddz/1  "ddz"
  Bus Selector5/2 -> Dynamic model/6(dy)  "<dy>"
  Bus Selector1/2 -> Rotation Matrix/2(q)  "<q>"
  Bus Selector1/3 -> Rotation Matrix/3(r)  "<r>"
  Discrete-Time Integrator/1 -> Scope6/1, Discrete-Time Integrator10/1, dy/1, Bus Creator3/4  "dy"
  Dynamic model/5(dq) -> Scope11/1, Discrete-Time Integrator4/1  "q"
  Dynamic model/4(dp) -> Scope10/1, Discrete-Time Integrator3/1  "p"
  Rotation Matrix/3(dpsi) -> Scope19/1, Discrete-Time Integrator8/1, Discrete Derivative2/1, Bus Creator3/12  "dpsi"
  Dynamic model/1(ddx) -> Discrete-Time Integrator1/1, Scope3/1, ddx/1  "ddx"
  Bus Selector/1 -> Dynamic model/2(phi)  "<roll_angle>"
  Bus Selector2/1 -> Dynamic model/8(p)  "<p>"
  Dynamic model/6(dr) -> Discrete-Time Integrator5/1  "r"
  Dynamic model/2(ddy) -> Discrete-Time Integrator/1, Scope4/1, ddy/1  "ddy"
  Bus Selector2/3 -> Dynamic model/10(r)  "<r>"
  In1/1 -> Dynamic model/1(channel)
  Bus Selector4/2 -> Rotation Matrix/5(theta)  "<pitch_angle>"
  Bus Selector5/3 -> Dynamic model/7(dz)  "<dz>"
  Bus Creator1/1 -> Bus Selector1/1, Bus Selector2/1
  Bus Selector/2 -> Dynamic model/3(theta)  "<pitch_angle>"
  Bus Selector/3 -> Dynamic model/4(psi)  "<yaw_angle>"
  Bus Selector1/1 -> Rotation Matrix/1(p)  "<p>"
  Bus Selector2/2 -> Dynamic model/9(q)  "<q>"
  Rotation Matrix/1(dphi) -> Scope17/1, Discrete-Time Integrator6/1, Bus Creator3/8, Discrete Derivative/1  "dphi"
  Discrete-Time Integrator1/1 -> Scope/1, Discrete-Time Integrator9/1, dx/1, Bus Creator3/2  "dx"
  Bus Creator3/1 -> State/1, Bus Selector4/1, Bus Selector5/1, Bus Selector/1
  Rotation Matrix/2(dtheta) -> Scope18/1, Discrete-Time Integrator7/1, Discrete Derivative1/1, Bus Creator3/10  "dtheta"
  Mux/1 -> Scope13/1
  des_x/1 -> Add/2, Mux/1
  Mux1/1 -> Scope13/2
  des_y/1 -> Add1/2, Mux1/1
  des_z/1 -> Add2/2, Mux2/1
  des_yaw/1 -> Add3/2, Mux3/1  "des_yaw"
  des_pitch/1 -> Mux4/1
  des_roll/1 -> Mux5/1
  Mux2/1 -> Scope13/3
  Mux3/1 -> Scope13/6
  Mux4/1 -> Scope13/4
  Mux5/1 -> Scope13/5
  Bus Creator/1 -> p q r/1
  Discrete-Time Integrator3/1 -> Scope8/1, Bus Creator/1, Discrete-Time Integrator12/1, Bus Creator1/1  "p"
  Discrete-Time Integrator4/1 -> Discrete-Time Integrator13/1, Scope9/1, Bus Creator/2, Bus Creator1/2  "q"
  Add/1 -> Abs/1
  Abs/1 -> Discrete-Time Integrator14/1
  Add3/1 -> Abs3/1
  Add1/1 -> Abs1/1
  Add2/1 -> Abs2/1
  Discrete-Time Integrator14/1 -> To Workspace3/1
  Abs1/1 -> Discrete-Time Integrator15/1
  Abs2/1 -> Discrete-Time Integrator17/1
  Abs3/1 -> Discrete-Time Integrator16/1
  disturbance_force_x/1 -> Dynamic model/11(d_f_x)
  disturbance_force_y/1 -> Dynamic model/12(d_f_y)
  disturbance_force_z/1 -> Dynamic model/13(d_f_z)
  disturbance_torque_p/1 -> Dynamic model/14(d_t_p)
  disturbance_torque_q/1 -> Dynamic model/15(d_t_q)
  disturbance_torque_r/1 -> Dynamic model/16(d_t_r)
  bias_x/1 -> Dynamic model/17(bias_x)
  bias_y/1 -> Dynamic model/18(bias_y)
  Discrete-Time Integrator5/1 -> Scope16/1, Bus Creator/3, Bus Creator1/3  "r"
  Discrete-Time Integrator6/1 -> Bus Creator3/7, To Workspace7/1, Mux5/2, Scope12/6, Scope2/1  "roll_angle"
  Discrete-Time Integrator7/1 -> Bus Creator3/9, To Workspace8/1, Mux4/2, Scope12/5, Scope2/2  "pitch_angle"
  Discrete-Time Integrator8/1 -> Bus Creator3/11, To Workspace9/1, Add3/1, Mux3/2, Scope12/4, Scope2/3  "yaw_angle"
  Discrete-Time Integrator9/1 -> To Workspace4/1, Scope1/1, Scope12/1, Add/1, Mux/2, Bus Creator3/1  "x"
  Discrete-Time Integrator10/1 -> To Workspace5/1, Scope12/2, Scope1/2, Add1/1, Mux1/2, Bus Creator3/3  "y"
  Discrete-Time Integrator11/1 -> To Workspace6/1, Scope1/3, Scope12/3, Add2/1, Mux2/2, Bus Creator3/5  "z"
  Discrete-Time Integrator12/1 -> Scope14/1
  Discrete-Time Integrator13/1 -> Scope15/1
  Discrete-Time Integrator15/1 -> To Workspace2/1
  Discrete-Time Integrator16/1 -> To Workspace/1
  Discrete-Time Integrator17/1 -> To Workspace1/1
  Discrete Derivative/1 -> Scope20/1, ddroll/1
  Discrete Derivative1/1 -> Scope21/1, ddpitch/1
  Discrete Derivative2/1 -> Scope22/1, ddyaw/1
  Dynamic model/10(u_4) -> Scope28/4, Bus Creator2/4
  Dynamic model/7(u_1) -> Scope28/1, Bus Creator2/1
  Dynamic model/8(u_2) -> Scope28/2, Bus Creator2/2
  Dynamic model/9(u_3) -> Scope28/3, Bus Creator2/3
  Bus Creator2/1 -> PropellerThrust/1

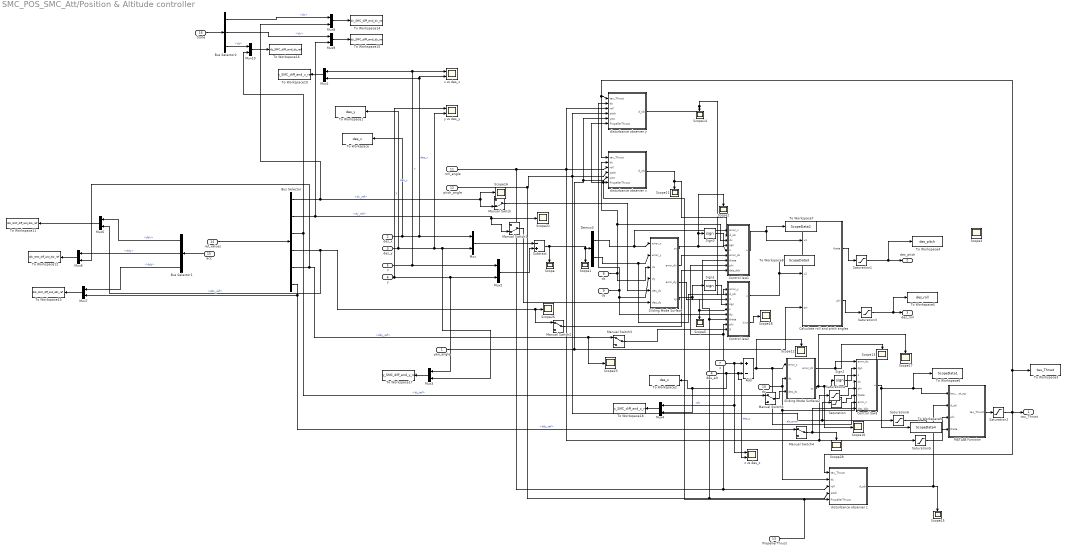
== system SMC_POS_SMC_Att/Position & Altitude controller ==
  yaw_angle : Inport
  des_x : Inport  Port=2
  des_y : Inport  Port=3
  des_alt : Inport  Port=4
  x : Inport  Port=5
  y : Inport  Port=6
  z : Inport  Port=7
  dx : Inport  Port=8
  dy : Inport  Port=9
  dz : Inport  Port=10
  roll_angle : Inport  Port=11
  pitch_angle : Inport  Port=12
  PropellerThrust : Inport  Port=13
  ref_values : Inport  Port=14
  acc : Inport  Port=15
  State : Inport  Port=16
  Add : Sum  Inputs=+-
  Bus Selector : BusSelector  OutputSignals=dx_ref,dy_ref,dz_ref,ddx_ref,ddy_ref,ddz_ref
  Bus Selector1 : BusSelector  OutputSignals=ddx,ddy,ddz
  Bus Selector2 : BusSelector  OutputSignals=dx,dy,dz
  "Calculate roll and pitch angles " : MATLAB Function  TreatAsAtomicUnit=on
  Control law1 : MATLAB Function  TreatAsAtomicUnit=on
  Control law2 : MATLAB Function  TreatAsAtomicUnit=on
  Control law3 : MATLAB Function  TreatAsAtomicUnit=on
  Demux3 : Demux  Outputs=2
  MATLAB Function : MATLAB Function  TreatAsAtomicUnit=on
  Manual Switch : ManualSwitch  CurrentSetting=0
  Manual Switch1 : ManualSwitch  CurrentSetting=0
  Manual Switch{2..5} (4 alike) : ManualSwitch
  Mux{,1..10} (11 alike) : Mux  Inputs=2
  Saturation{,4..6} (4 alike) : Saturate  UpperLimit=1.5  LowerLimit=-1.5
  Saturation1 : Saturate  UpperLimit=0.8727  LowerLimit=-0.8727
  Saturation2 : Saturate  UpperLimit=2  LowerLimit=1
  Saturation3 : Saturate  UpperLimit=0.8727  LowerLimit=-0.8727
  Scope{,1..3,5,10..18,21,23,26,28} (18 alike) : Scope
  Sign1 : Signum  ZeroCross=off
  Sign2 : Signum  ZeroCross=off
  Sign3 : Signum  ZeroCross=off
  Sliding Mode Surface : MATLAB Function  TreatAsAtomicUnit=on
  Sliding Mode Surface2 : MATLAB Function  TreatAsAtomicUnit=on
  Subtract : Sum  Inputs=-+
  To Workspace : ToWorkspace  VariableName=des_x  SampleTime=-1
      settings: Save2DSignal=2-D array (concatenate along first dimension)
  To Workspace1 : ToWorkspace  VariableName=des_y  SampleTime=-1
      settings: Save2DSignal=2-D array (concatenate along first dimension)
  To Workspace10 : ToWorkspace  VariableName=x_SMC_diff_and_x_ref  SaveFormat=Timeseries  SampleTime=-1
  To Workspace11 : ToWorkspace  VariableName=ddx_SMC_diff_and_ddx_ref  SaveFormat=Timeseries  SampleTime=-1
  To Workspace12 : ToWorkspace  VariableName=ddy_SMC_diff_and_ddy_ref  SaveFormat=Timeseries  SampleTime=-1
  To Workspace13 : ToWorkspace  VariableName=ddz_SMC_diff_and_ddz_ref  SaveFormat=Timeseries  SampleTime=-1
  To Workspace14 : ToWorkspace  VariableName=dx_SMC_diff_and_dx_ref  SaveFormat=Timeseries  SampleTime=-1
  To Workspace15 : ToWorkspace  VariableName=dy_SMC_diff_and_dy_ref  SaveFormat=Timeseries  SampleTime=-1
  To Workspace16 : ToWorkspace  VariableName=dz_SMC_diff_and_dz_ref  SaveFormat=Timeseries  SampleTime=-1
  To Workspace17 : ToWorkspace  VariableName=y_SMC_diff_and_y_ref  SaveFormat=Timeseries  SampleTime=-1
  To Workspace18 : ToWorkspace  VariableName=z_SMC_diff_and_z_ref  SaveFormat=Timeseries  SampleTime=-1
  To Workspace2 : ToWorkspace  VariableName=des_z  SampleTime=-1
      settings: Save2DSignal=2-D array (concatenate along first dimension)
  To Workspace3 : ToWorkspace  VariableName=tau_Thrust  SampleTime=-1
      settings: Save2DSignal=2-D array (concatenate along first dimension)
  To Workspace4 : ToWorkspace  VariableName=des_pitch  SampleTime=-1
      settings: Save2DSignal=2-D array (concatenate along first dimension)
  To Workspace5 : ToWorkspace  VariableName=des_roll  SampleTime=-1
      settings: Save2DSignal=2-D array (concatenate along first dimension)
  To Workspace6 : ToWorkspace  VariableName=ScopeData1  SampleTime=-1
      settings: Save2DSignal=2-D array (concatenate along first dimension)
  To Workspace7 : ToWorkspace  VariableName=ScopeData2  SampleTime=-1
      settings: Save2DSignal=2-D array (concatenate along first dimension)
  To Workspace8 : ToWorkspace  VariableName=ScopeData3  SampleTime=-1
      settings: Save2DSignal=2-D array (concatenate along first dimension)
  To Workspace9 : ToWorkspace  VariableName=ScopeData4  SampleTime=-1
      settings: Save2DSignal=2-D array (concatenate along first dimension)
  disturbance observer x : Subsystem
  disturbance observer y : Subsystem
  disturbance observer z : Subsystem
  x vs des_x : Scope  NumInputPorts=2
  y vs des_y : Scope  NumInputPorts=2
  z vs des_z : Scope  NumInputPorts=2
  tau_Thrust : Outport
  des_pitch : Outport  Port=2
  des_roll : Outport  Port=3
  wires:
  Sign3/1 -> Control law1/4(sgn)
  Sliding Mode Surface/2(error_dx) -> Control law1/6(error_dx)
  Sliding Mode Surface/3(error_dy) -> Control law2/3(error_dy)
  Sign1/1 -> Control law2/4(sgn)
  Subtract/1 -> Scope1/1, Demux3/1, Scope/1
  Mux/1 -> Subtract/1
  Mux2/1 -> Subtract/2
  Demux3/1 -> Control law1/1(error_x), Sliding Mode Surface/1(error_x)
  Demux3/2 -> Control law2/1(error_y), Sliding Mode Surface/2(error_y)
  dx/1 -> disturbance observer x/2(dx), Control law1/3(dx), Sliding Mode Surface/3(dx)
  dy/1 -> disturbance observer y/2(dy), Control law2/6(dy), Sliding Mode Surface/4(dy)
  yaw_angle/1 -> "Calculate roll and pitch angles "/3(psi), disturbance observer y/5(yaw), disturbance observer x/5(yaw)
  "Calculate roll and pitch angles "/1(theta) -> Saturation1/1
  "Calculate roll and pitch angles "/2(phi) -> Saturation3/1
  Sliding Mode Surface2/2(sz) -> Scope17/1, Scope10/1, Sign2/1, Control law3/3(s)
  Sliding Mode Surface2/1(error_dz) -> Scope13/1, Control law3/1(error_dz)
  Sign2/1 -> Control law3/2(sgn)
  dz/1 -> disturbance observer z/2(dz), Control law3/4(dz), Sliding Mode Surface2/2(dz)
  Add/1 -> Control law3/7(error_z), Sliding Mode Surface2/1(error_z), Scope12/1  "alt_error"
  Saturation3/1 -> To Workspace5/1, des_roll/1
  Saturation1/1 -> To Workspace4/1, des_pitch/1
  Sliding Mode Surface/1(sx) -> Scope2/1, Sign3/1, Control law1/5(s)
  Sliding Mode Surface/4(sy) -> Control law2/5(s), Scope5/1, Sign1/1
  roll_angle/1 -> disturbance observer z/3("roll "), Control law2/8(phi), Control law1/8(phi), Saturation5/1, Saturation4/1, disturbance observer x/3("roll "), disturbance observer y/3("roll ")
  pitch_angle/1 -> disturbance observer z/4(pitch), Control law1/7(theta), Control law2/7(theta), Saturation6/1, Saturation/1, disturbance observer x/4(pitch), disturbance observer y/4(pitch)
  disturbance observer x/1(d_ob) -> Control law1/2(d_ob), Scope11/1
  disturbance observer y/1(d_ob) -> Control law2/2(d_ob), Scope14/1
  disturbance observer z/1(d_ob) -> MATLAB Function/2(d_ob), Scope15/1
  MATLAB Function/1(tau_Thrust) -> Saturation2/1
  Saturation2/1 -> disturbance observer z/1(tau_Thrust), To Workspace3/1, disturbance observer x/1(tau_Thrust), disturbance observer y/1(tau_Thrust), tau_Thrust/1
  Control law3/1(u) -> To Workspace9/1, To Workspace6/1, MATLAB Function/1(tau_Thrust_og)
  Control law2/2(kint) -> Scope18/1
  Saturation/1 -> Control law3/6(theta)
  Saturation4/1 -> Control law3/5(phi)
  Control law1/1(u) -> To Workspace7/1, "Calculate roll and pitch angles "/1(u1)
  Control law2/1(u) -> To Workspace8/1, "Calculate roll and pitch angles "/2(u2)
  des_x/1 -> To Workspace/1, x vs des_x/2, Mux1/2, Mux/1  "des_x"
  Manual Switch/1 -> Sliding Mode Surface/5(des_dx)
  Manual Switch1/1 -> Sliding Mode Surface/6(des_dy)
  Manual Switch2/1 -> Control law1/9(des_ddx)
  Manual Switch3/1 -> Control law2/9(des_ddy)
  Manual Switch4/1 -> Scope28/1, Control law3/8(des_ddz)
  Saturation5/1 -> MATLAB Function/3(phi)
  Saturation6/1 -> MATLAB Function/4(theta)
  Manual Switch5/1 -> Sliding Mode Surface2/3(des_dz)
  PropellerThrust/1 -> disturbance observer y/6(PropellerThrust), disturbance observer x/6(PropellerThrust), disturbance observer z/5(PropellerThrust)
  ref_values/1 -> Bus Selector/1
  Bus Selector/2 -> Mux9/2, Manual Switch1/2, Scope21/1  "<dy_ref>"
  Bus Selector2/1 -> Mux8/1  "<dx>"
  Bus Selector/4 -> Mux5/2, Manual Switch2/1, Scope26/1  "<ddx_ref>"
  Bus Selector2/2 -> Mux9/1  "<dy>"
  x/1 -> Mux2/1, x vs des_x/1, Mux1/1  "x"
  acc/1 -> Bus Selector1/1
  Mux8/1 -> To Workspace14/1
  State/1 -> Bus Selector2/1
  Bus Selector/6 -> Mux7/2, Manual Switch4/1  "<ddz_ref>"
  Mux9/1 -> To Workspace15/1
  Bus Selector/3 -> Mux10/2, Manual Switch5/1  "<dz_ref>"
  Bus Selector1/3 -> Mux7/1  "<ddz>"
  Mux10/1 -> To Workspace16/1
  Bus Selector/5 -> Scope23/1, Manual Switch3/1, Mux6/2  "<ddy_ref>"
  Bus Selector/1 -> Mux8/2, Manual Switch/2, Scope16/1  "<dx_ref>"
  Bus Selector1/1 -> Mux5/1  "<ddx>"
  Mux7/1 -> To Workspace13/1
  Bus Selector2/3 -> Mux10/1  "<dz>"
  Bus Selector1/2 -> Mux6/1  "<ddy>"
  Mux1/1 -> To Workspace10/1
  Mux5/1 -> To Workspace11/1
  Mux6/1 -> To Workspace12/1
  Mux4/1 -> To Workspace18/1
  y/1 -> y vs des_y/1, Mux3/1, Mux2/2  "y"
  Mux3/1 -> To Workspace17/1
  des_y/1 -> To Workspace1/1, Mux3/2, Mux/2, y vs des_y/2  "des_y"
  des_alt/1 -> Mux4/2, To Workspace2/1, z vs des_z/2, Add/2  "des_z"
  z/1 -> z vs des_z/1, Mux4/1, Add/1  "alt"

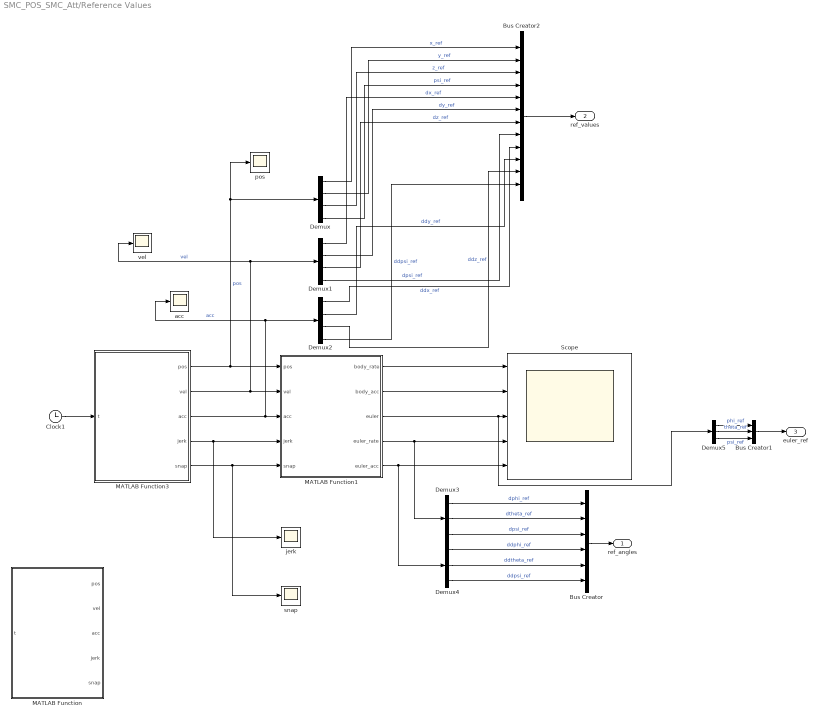
== system SMC_POS_SMC_Att/Reference Values ==
  Bus Creator : BusCreator  Inputs=6
  Bus Creator1 : BusCreator  Inputs=3
  Bus Creator2 : BusCreator  Inputs=12
  Clock1 : Clock
  Demux : Demux
  Demux1 : Demux
  Demux2 : Demux
  Demux3 : Demux  Outputs=3
  Demux4 : Demux  Outputs=3
  Demux5 : Demux  Outputs=3
  MATLAB Function : MATLAB Function  TreatAsAtomicUnit=on
  MATLAB Function1 : MATLAB Function  TreatAsAtomicUnit=on
  MATLAB Function3 : MATLAB Function  TreatAsAtomicUnit=on
  Scope : Scope  NumInputPorts=5
  acc : Scope
  jerk : Scope
  pos : Scope
  snap : Scope
  vel : Scope
  ref_angles : Outport
  ref_values : Outport  Port=2
  euler_ref : Outport  Port=3
  wires:
  MATLAB Function1/3(euler) -> Demux5/1, Scope/3
  MATLAB Function1/5(euler_acc) -> Scope/5, Demux4/1
  Clock1/1 -> MATLAB Function3/1(t)
  MATLAB Function1/1(body_rate) -> Scope/1
  MATLAB Function3/4(jerk) -> jerk/1, MATLAB Function1/4(jerk)
  MATLAB Function1/4(euler_rate) -> Scope/4, Demux3/1
  MATLAB Function3/2(vel) -> vel/1, Demux1/1, MATLAB Function1/2(vel)  "vel"
  MATLAB Function3/5(snap) -> snap/1, MATLAB Function1/5(snap)
  MATLAB Function3/3(acc) -> MATLAB Function1/3(acc), acc/1, Demux2/1  "acc"
  MATLAB Function3/1(pos) -> Demux/1, pos/1, MATLAB Function1/1(pos)  "pos"
  MATLAB Function1/2(body_acc) -> Scope/2
  Demux3/1 -> Bus Creator/1  "dphi_ref"
  Demux3/2 -> Bus Creator/2  "dtheta_ref"
  Demux/1 -> Bus Creator2/1  "x_ref"
  Demux/2 -> Bus Creator2/2  "y_ref"
  Demux/3 -> Bus Creator2/3  "z_ref"
  Demux/4 -> Bus Creator2/4  "psi_ref"
  Demux1/1 -> Bus Creator2/5  "dx_ref"
  Demux1/2 -> Bus Creator2/6  "dy_ref"
  Demux1/3 -> Bus Creator2/7  "dz_ref"
  Demux1/4 -> Bus Creator2/8  "dpsi_ref"
  Demux2/1 -> Bus Creator2/9  "ddx_ref"
  Demux2/2 -> Bus Creator2/10  "ddy_ref"
  Demux2/3 -> Bus Creator2/11  "ddz_ref"
  Demux2/4 -> Bus Creator2/12  "ddpsi_ref"
  Demux3/3 -> Bus Creator/3  "dpsi_ref"
  Demux4/1 -> Bus Creator/4  "ddphi_ref"
  Demux4/3 -> Bus Creator/6  "ddpsi_ref"
  Demux4/2 -> Bus Creator/5  "ddtheta_ref"
  Bus Creator/1 -> ref_angles/1
  Bus Creator2/1 -> ref_values/1
  Demux5/1 -> Bus Creator1/1  "phi_ref"
  Demux5/2 -> Bus Creator1/2  "theta_ref"
  Demux5/3 -> Bus Creator1/3  "psi_ref"
  Bus Creator1/1 -> euler_ref/1

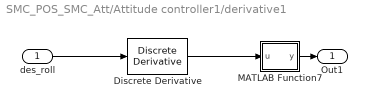
== system SMC_POS_SMC_Att/Attitude controller1/derivative1 ==
  des_roll : Inport
  Discrete Derivative : simulink/Discrete/Discrete Derivative  gainval=1.0  ICPrevScaledInput=0.0  OutMin=[]  OutMax=[]  OutDataType=fixdt(1, 16)  OutScaling=2^-10  DoSatur=off
  MATLAB Function7 : MATLAB Function  TreatAsAtomicUnit=on
  Out1 : Outport
  wires:
  des_roll/1 -> Discrete Derivative/1
  MATLAB Function7/1(y) -> Out1/1
  Discrete Derivative/1 -> MATLAB Function7/1(u)

== system SMC_POS_SMC_Att/Attitude controller1/derivative10 ==
  des_roll : Inport
  Discrete Derivative : simulink/Discrete/Discrete Derivative  gainval=1.0  ICPrevScaledInput=0.0  OutMin=[]  OutMax=[]  OutDataType=fixdt(1, 16)  OutScaling=2^-10  DoSatur=off
  MATLAB Function7 : MATLAB Function  TreatAsAtomicUnit=on
  Out1 : Outport
  wires:
  des_roll/1 -> Discrete Derivative/1
  MATLAB Function7/1(y) -> Out1/1
  Discrete Derivative/1 -> MATLAB Function7/1(u)

== system SMC_POS_SMC_Att/Attitude controller1/derivative2 ==
  des_roll : Inport
  Discrete Derivative : simulink/Discrete/Discrete Derivative  gainval=1.0  ICPrevScaledInput=0.0  OutMin=[]  OutMax=[]  OutDataType=fixdt(1, 16)  OutScaling=2^-10  DoSatur=off
  MATLAB Function7 : MATLAB Function  TreatAsAtomicUnit=on
  Out1 : Outport
  wires:
  des_roll/1 -> Discrete Derivative/1
  MATLAB Function7/1(y) -> Out1/1
  Discrete Derivative/1 -> MATLAB Function7/1(u)

== system SMC_POS_SMC_Att/Attitude controller1/derivative3 ==
  des_roll : Inport
  Discrete Derivative : simulink/Discrete/Discrete Derivative  gainval=1.0  ICPrevScaledInput=0.0  OutMin=[]  OutMax=[]  OutDataType=fixdt(1, 16)  OutScaling=2^-10  DoSatur=off
  MATLAB Function7 : MATLAB Function  TreatAsAtomicUnit=on
  Out1 : Outport
  wires:
  des_roll/1 -> Discrete Derivative/1
  MATLAB Function7/1(y) -> Out1/1
  Discrete Derivative/1 -> MATLAB Function7/1(u)

== system SMC_POS_SMC_Att/Attitude controller1/derivative4 ==
  In1 : Inport
  Discrete Derivative : simulink/Discrete/Discrete Derivative  gainval=1.0  ICPrevScaledInput=0.0  OutMin=[]  OutMax=[]  OutDataType=fixdt(1, 16)  OutScaling=2^-10  DoSatur=off
  MATLAB Function7 : MATLAB Function  TreatAsAtomicUnit=on
  Out1 : Outport
  wires:
  In1/1 -> Discrete Derivative/1
  MATLAB Function7/1(y) -> Out1/1
  Discrete Derivative/1 -> MATLAB Function7/1(u)

== system SMC_POS_SMC_Att/Attitude controller1/derivative5 ==
  In1 : Inport
  Discrete Derivative : simulink/Discrete/Discrete Derivative  gainval=1.0  ICPrevScaledInput=0.0  OutMin=[]  OutMax=[]  OutDataType=fixdt(1, 16)  OutScaling=2^-10  DoSatur=off
  MATLAB Function7 : MATLAB Function  TreatAsAtomicUnit=on
  Out1 : Outport
  wires:
  In1/1 -> Discrete Derivative/1
  MATLAB Function7/1(y) -> Out1/1
  Discrete Derivative/1 -> MATLAB Function7/1(u)

== system SMC_POS_SMC_Att/Attitude controller1/derivative6 ==
  In1 : Inport
  Discrete Derivative : simulink/Discrete/Discrete Derivative  gainval=1.0  ICPrevScaledInput=0.0  OutMin=[]  OutMax=[]  OutDataType=fixdt(1, 16)  OutScaling=2^-10  DoSatur=off
  MATLAB Function7 : MATLAB Function  TreatAsAtomicUnit=on
  Out1 : Outport
  wires:
  In1/1 -> Discrete Derivative/1
  MATLAB Function7/1(y) -> Out1/1
  Discrete Derivative/1 -> MATLAB Function7/1(u)

== system SMC_POS_SMC_Att/Attitude controller1/derivative7 ==
  In1 : Inport
  Discrete Derivative : simulink/Discrete/Discrete Derivative  gainval=1.0  ICPrevScaledInput=0.0  OutMin=[]  OutMax=[]  OutDataType=fixdt(1, 16)  OutScaling=2^-10  DoSatur=off
  MATLAB Function7 : MATLAB Function  TreatAsAtomicUnit=on
  Out1 : Outport
  wires:
  In1/1 -> Discrete Derivative/1
  MATLAB Function7/1(y) -> Out1/1
  Discrete Derivative/1 -> MATLAB Function7/1(u)

== system SMC_POS_SMC_Att/Attitude controller1/derivative8 ==
  In1 : Inport
  Discrete Derivative : simulink/Discrete/Discrete Derivative  gainval=1.0  ICPrevScaledInput=0.0  OutMin=[]  OutMax=[]  OutDataType=fixdt(1, 16)  OutScaling=2^-10  DoSatur=off
  MATLAB Function7 : MATLAB Function  TreatAsAtomicUnit=on
  Out1 : Outport
  wires:
  In1/1 -> Discrete Derivative/1
  MATLAB Function7/1(y) -> Out1/1
  Discrete Derivative/1 -> MATLAB Function7/1(u)

== system SMC_POS_SMC_Att/Attitude controller1/derivative9 ==
  In1 : Inport
  Discrete Derivative : simulink/Discrete/Discrete Derivative  gainval=1.0  ICPrevScaledInput=0.0  OutMin=[]  OutMax=[]  OutDataType=fixdt(1, 16)  OutScaling=2^-10  DoSatur=off
  MATLAB Function7 : MATLAB Function  TreatAsAtomicUnit=on
  Out1 : Outport
  wires:
  In1/1 -> Discrete Derivative/1
  MATLAB Function7/1(y) -> Out1/1
  Discrete Derivative/1 -> MATLAB Function7/1(u)
